simulink model "test_fft"  (R2012b)
settings: Solver=ode45  StartTime=0.0  StopTime=10.0  RelTol=1e-3
libraries: xbsIndex_r4 x6538, casper_library_misc x220, casper_library_delays x31, xbsReplacements_r4 x4, casper_library_ffts_twiddle x2, simulink x1
(part 88 of 104)

== system test_fft/fft0/fft_biplex_real_4x0/biplex_core/fft_stage_12/butterfly_direct/twiddle_general_4mult/coeff_gen ==
  rst : Inport
  Counter : xbsIndex_r4/Counter  cnt_type=Free Running  cnt_to=Inf  operation=Up  start_count=0  cnt_by_val=1  arith_type=Unsigned  n_bits=11  bin_pt=0  load_pin=off  rst=on  en=off  explicit_period=on  period=1  dbl_ovrd=off  use_behavioral_HDL=off  implementation=Fabric  block_type=counter
  ROM : xbsIndex_r4/ROM  depth=2048  initVector="[1                                      0                     0.7071075439453125                    -0.7071075439453125                     0.9238739013671875                       -0.3826904296875                        0.3826904296875                    -0.9238739013671875                     0.9807891845703125                    -0.1950836181640625                      0.555572509765625                    -0.8314666748046875                     0.8314666748046875                     -0.555572509765625                     0.1950836181640625                    -0.9807891845703125                       0.99517822265625                       -0.0980224609375                        0.6343994140625                      -0.77301025390625                      0.881927490234375                    -0.4713897705078125                         0.290283203125                     -0.956939697265625                      0.956939697265625                        -0.290283203125                     0.4713897705078125                     -0.881927490234375                       0.77301025390625                       -0.6343994140625                        0.0980224609375                      -0.99517822265625                     0.9987945556640625                        -0.049072265625                     0.6715545654296875                    -0.7409515380859375                       0.90399169921875                      -0.42755126953125                      0.336883544921875                    -0.9415435791015625                       0.97003173828125                      -0.24298095703125                       0.51409912109375                      -0.85772705078125                     0.8032073974609375                           -0.595703125                         0.146728515625                    -0.9891815185546875                     0.9891815185546875                        -0.146728515625                            0.595703125                    -0.8032073974609375                       0.85772705078125                      -0.51409912109375                       0.24298095703125                      -0.97003173828125                     0.9415435791015625                     -0.336883544921875                       0.42755126953125                      -0.90399169921875                     0.7409515380859375                    -0.6715545654296875                         0.049072265625                    -0.9987945556640625                       0.99969482421875                       -0.0245361328125                      0.689544677734375                       -0.7242431640625                      0.914215087890625                     -0.405242919921875                      0.359893798828125                    -0.9329986572265625                        0.9757080078125                    -0.2191009521484375                      0.535003662109375                       -0.8448486328125                     0.8175811767578125                       -0.5758056640625                       0.17095947265625                    -0.9852752685546875                     0.9924774169921875                     -0.122406005859375                            0.615234375                    -0.7883453369140625                      0.870086669921875                    -0.4929046630859375                     0.2667083740234375                     -0.963775634765625                       0.94952392578125                    -0.3136749267578125                      0.449615478515625                     -0.893218994140625                        0.7572021484375                     -0.653167724609375                     0.0735626220703125                     -0.997283935546875                      0.997283935546875                    -0.0735626220703125                      0.653167724609375                       -0.7572021484375                      0.893218994140625                     -0.449615478515625                     0.3136749267578125 ...(+75836 chars)]"  distributed_mem=Block RAM  rst=off  init_reg=0  en=off  latency=4  gui_display_data_type=Fixed-point  arith_type="Signed  (2's comp)"  n_bits=18  bin_pt=16  preci_type=Single  exp_width=8  frac_width=24  dbl_ovrd=off  optimize=Area  use_rpm=on  block_type=sprom
  ROM1 : xbsIndex_r4/ROM  depth=2048  initVector="[0                                     -1                    -0.7071075439453125                    -0.7071075439453125                       -0.3826904296875                    -0.9238739013671875                    -0.9238739013671875                       -0.3826904296875                    -0.1950836181640625                    -0.9807891845703125                    -0.8314666748046875                     -0.555572509765625                     -0.555572509765625                    -0.8314666748046875                    -0.9807891845703125                    -0.1950836181640625                       -0.0980224609375                      -0.99517822265625                      -0.77301025390625                       -0.6343994140625                    -0.4713897705078125                     -0.881927490234375                     -0.956939697265625                        -0.290283203125                        -0.290283203125                     -0.956939697265625                     -0.881927490234375                    -0.4713897705078125                       -0.6343994140625                      -0.77301025390625                      -0.99517822265625                       -0.0980224609375                        -0.049072265625                    -0.9987945556640625                    -0.7409515380859375                    -0.6715545654296875                      -0.42755126953125                      -0.90399169921875                    -0.9415435791015625                     -0.336883544921875                      -0.24298095703125                      -0.97003173828125                      -0.85772705078125                      -0.51409912109375                           -0.595703125                    -0.8032073974609375                    -0.9891815185546875                        -0.146728515625                        -0.146728515625                    -0.9891815185546875                    -0.8032073974609375                           -0.595703125                      -0.51409912109375                      -0.85772705078125                      -0.97003173828125                      -0.24298095703125                     -0.336883544921875                    -0.9415435791015625                      -0.90399169921875                      -0.42755126953125                    -0.6715545654296875                    -0.7409515380859375                    -0.9987945556640625                        -0.049072265625                       -0.0245361328125                      -0.99969482421875                       -0.7242431640625                     -0.689544677734375                     -0.405242919921875                     -0.914215087890625                    -0.9329986572265625                     -0.359893798828125                    -0.2191009521484375                       -0.9757080078125                       -0.8448486328125                     -0.535003662109375                       -0.5758056640625                    -0.8175811767578125                    -0.9852752685546875                      -0.17095947265625                     -0.122406005859375                    -0.9924774169921875                    -0.7883453369140625                           -0.615234375                    -0.4929046630859375                     -0.870086669921875                     -0.963775634765625                    -0.2667083740234375                    -0.3136749267578125                      -0.94952392578125                     -0.893218994140625                     -0.449615478515625                     -0.653167724609375                       -0.7572021484375                     -0.997283935546875                    -0.0735626220703125                    -0.0735626220703125                     -0.997283935546875                       -0.7572021484375                     -0.653167724609375                     -0.449615478515625                     -0.893218994140625                      -0.94952392578125 ...(+75836 chars)]"  distributed_mem=Block RAM  rst=off  init_reg=0  en=off  latency=4  gui_display_data_type=Fixed-point  arith_type="Signed  (2's comp)"  n_bits=18  bin_pt=16  preci_type=Single  exp_width=8  frac_width=24  dbl_ovrd=off  optimize=Area  use_rpm=on  block_type=sprom
  Slice : xbsIndex_r4/Slice  nbits=11  boolean_output=off  mode=Upper Bit Location + Width  bit1=0  base1=MSB of Input  bit0=0  base0=LSB of Input  dbl_ovrd=off  block_type=slice
  ri_to_c : casper_library_misc/ri_to_c
  w : Outport
  wires:
  ri_to_c/1 -> w/1
  rst/1 -> Counter/1
  Counter/1 -> Slice/1
  Slice/1 -> ROM/1, ROM1/1
  ROM/1 -> ri_to_c/1
  ROM1/1 -> ri_to_c/2
